simulink library "halin"  (R2021b)
settings: Solver=VariableStepAuto  StartTime=0.0  StopTime=10.0  RelTol=1e-3
undefined symbols (not defined in the file): KHAL_CAN1ABM1E2E_flg, KHAL_CAN1ESC1E2E_flg, KHAL_CAN1ESC5E2E_flg, KHAL_CAN1ESC7E2E_flg, KHAL_CAN1FCM2E2E_flg, KHAL_CAN1FCM3E2E_flg, KHAL_CAN1FCM4E2E_flg, KHAL_CAN3BMS1E2E_flg, KHAL_CAN3BMS6E2E_flg, KHAL_CAN3CCU1E2E_flg, KHAL_CAN3CCU2E2E_flg, KHAL_CAN3MCUF1E2E_flg, KHAL_CAN3MCUR1E2E_flg, KHAL_CAN3Shifter1E2E_flg, TRUE
libraries: simulink x420, FVT_lib x149, hcu_lib x49
(part 5 of 14)

== system halin/HAL_IN/CAN1/ESC1 ==
  DT_CAN1_SG_ESC1 : Inport
  0x5f : Constant  Value=0x5f
  0xb3 : Constant  Value=0xb3
  BitwiseAND{,1..9} (10 alike) : simulink/Logic and Bit Operations/Bitwise Operator  logicop=AND  UseBitMask=on  BitMask=0xFF  BitMaskRealWorld=Stored Integer
  BitwiseOR : simulink/Logic and Bit Operations/Bitwise Operator  logicop=OR  UseBitMask=off  NumInputPorts=2  BitMask=bin2dec('11011001')  BitMaskRealWorld=Stored Integer
  BitwiseOR1 : simulink/Logic and Bit Operations/Bitwise Operator  logicop=OR  UseBitMask=off  NumInputPorts=3  BitMask=bin2dec('11011001')  BitMaskRealWorld=Stored Integer
  BitwiseOR{2..6} (5 alike) : simulink/Logic and Bit Operations/Bitwise Operator  logicop=OR  UseBitMask=off  BitMask=bin2dec('11011001')  BitMaskRealWorld=Stored Integer
  DDM_ESC_CS&RC_Comparison : FVT_lib/hal/DDM_ESC_CS&RC_Comparison  MsgCycleTime=10
  Data Type Conversion{,1..9} (10 alike) : DataTypeConversion  OutDataTypeStr=uint8
  ESC1CS : Subsystem
  ESC1RC : Subsystem
  FrPTCSActive : Subsystem
  FrntAxlTrqReqDrv : Subsystem
  KHAL_CAN1ESC1E2E_flg : Constant  Value=KHAL_CAN1ESC1E2E_flg
  LeftShift : ArithShift  BitShiftNumber=4  BitShiftDirection=Left
  LeftShift1 : ArithShift  BitShiftDirection=Left
  LeftShift2 : ArithShift  BitShiftNumber=5  BitShiftDirection=Left
  LeftShift3 : ArithShift  BitShiftNumber=6  BitShiftDirection=Left
  MessageRollingCounter : FVT_lib/hal/MessageRollingCounter  CounterMAX=14  task_time_ms=5  msg_time_ms=10
  Mux : Mux  Inputs=8
  RearAxlTrqReqDrv : Subsystem
  RightShift : ArithShift  BitShiftNumber=8
  RightShift1 : ArithShift
  RightShift2 : ArithShift  BitShiftNumber=8
  RightShift3 : ArithShift
  RightShift4 : ArithShift  BitShiftNumber=8
  RightShift5 : ArithShift
  RrPTCSActive : Subsystem
  VehSpeed : Subsystem
  bus_selector : BusSelector  OutputSignals=CAN1_ESC1_CS,CAN1_ESC1_RC,CAN1_Fr_PTCS_Active,CAN1_FrntAxlTrqReq_Drv,CAN1_RearAxlTrqReq_Drv,CAN1_Rr_PTCS_Active,CAN1_VehSpeed
  bus_selector1 : BusSelector  OutputSignals=CAN1_ESC1_CS
  bus_selector2 : BusSelector  OutputSignals=CAN1_ESC1_RC
  bus_selector3 : BusSelector  OutputSignals=CAN1_Fr_PTCS_Active
  bus_selector4 : BusSelector  OutputSignals=CAN1_FrntAxlTrqReq_Drv
  bus_selector5 : BusSelector  OutputSignals=CAN1_RearAxlTrqReq_Drv
  bus_selector6 : BusSelector  OutputSignals=CAN1_Rr_PTCS_Active
  bus_selector7 : BusSelector  OutputSignals=CAN1_VehSpeed
  constant : Constant  Value=0x0  OutDataTypeStr=uint8
  VHAL_ESC1CSErr_flg : Outport
  VHAL_ESC1RCErr_flg : Outport  Port=2
  VHAL_ESC1CS_enum : Outport  Port=3
  VHAL_ESC1RC_enum : Outport  Port=4
  VHAL_FrPTCSActive_flg : Outport  Port=5
  VHAL_FrntAxlTrqReqDrv_Nm : Outport  Port=6
  VHAL_RearAxlTrqReqDrv_Nm : Outport  Port=7
  VHAL_RrPTCSActive_flg : Outport  Port=8
  VHAL_VehSpeed_kph : Outport  Port=9
  wires:
  DT_CAN1_SG_ESC1/1 -> [DT_CAN1_SG_ESC1]
  [DT_CAN1_SG_ESC1] -> bus_selector/1
  bus_selector/1 -> [CAN1_ESC1_CS]  "<CAN1_ESC1_CS>"
  [CAN1_ESC1_CS] -> LeftShift/1
  LeftShift/1 -> BitwiseAND/1
  BitwiseAND/1 -> [Byte_0_CAN1_ESC1_CS]
  bus_selector/2 -> [CAN1_ESC1_RC]  "<CAN1_ESC1_RC>"
  [CAN1_ESC1_RC] -> LeftShift1/1
  LeftShift1/1 -> BitwiseAND1/1
  BitwiseAND1/1 -> [Byte_0_CAN1_ESC1_RC]
  bus_selector/3 -> [CAN1_Fr_PTCS_Active]  "<CAN1_Fr_PTCS_Active>"
  [CAN1_Fr_PTCS_Active] -> LeftShift2/1
  LeftShift2/1 -> BitwiseAND2/1
  BitwiseAND2/1 -> [Byte_2_CAN1_Fr_PTCS_Active]
  bus_selector/4 -> [CAN1_FrntAxlTrqReq_Drv]  "<CAN1_FrntAxlTrqReq_Drv>"
  [CAN1_FrntAxlTrqReq_Drv] -> RightShift/1, RightShift1/1
  RightShift/1 -> BitwiseAND3/1
  BitwiseAND3/1 -> [Byte_4_CAN1_FrntAxlTrqReq_Drv]
  RightShift1/1 -> BitwiseAND4/1
  BitwiseAND4/1 -> [Byte_5_CAN1_FrntAxlTrqReq_Drv]
  bus_selector/5 -> [CAN1_RearAxlTrqReq_Drv]  "<CAN1_RearAxlTrqReq_Drv>"
  [CAN1_RearAxlTrqReq_Drv] -> RightShift2/1, RightShift3/1
  RightShift2/1 -> BitwiseAND5/1
  BitwiseAND5/1 -> [Byte_6_CAN1_RearAxlTrqReq_Drv]
  RightShift3/1 -> BitwiseAND6/1
  BitwiseAND6/1 -> [Byte_7_CAN1_RearAxlTrqReq_Drv]
  bus_selector/6 -> [CAN1_Rr_PTCS_Active]  "<CAN1_Rr_PTCS_Active>"
  [CAN1_Rr_PTCS_Active] -> LeftShift3/1
  LeftShift3/1 -> BitwiseAND7/1
  BitwiseAND7/1 -> [Byte_2_CAN1_Rr_PTCS_Active]
  bus_selector/7 -> [CAN1_VehSpeed]  "<CAN1_VehSpeed>"
  [CAN1_VehSpeed] -> RightShift4/1, RightShift5/1
  RightShift4/1 -> BitwiseAND8/1
  BitwiseAND8/1 -> [Byte_2_CAN1_VehSpeed]
  RightShift5/1 -> BitwiseAND9/1
  BitwiseAND9/1 -> [Byte_3_CAN1_VehSpeed]
  Data Type Conversion/1 -> BitwiseOR/1
  [Byte_0_CAN1_ESC1_CS] -> Data Type Conversion/1
  Data Type Conversion1/1 -> BitwiseOR/2
  [Byte_0_CAN1_ESC1_RC] -> Data Type Conversion1/1
  BitwiseOR/1 -> [Byte_0]
  constant/1 -> [Byte_1]
  Data Type Conversion2/1 -> BitwiseOR1/1
  [Byte_2_CAN1_Fr_PTCS_Active] -> Data Type Conversion2/1
  Data Type Conversion3/1 -> BitwiseOR1/2
  [Byte_2_CAN1_Rr_PTCS_Active] -> Data Type Conversion3/1
  Data Type Conversion4/1 -> BitwiseOR1/3
  [Byte_2_CAN1_VehSpeed] -> Data Type Conversion4/1
  BitwiseOR1/1 -> [Byte_2]
  Data Type Conversion5/1 -> BitwiseOR2/1
  [Byte_3_CAN1_VehSpeed] -> Data Type Conversion5/1
  BitwiseOR2/1 -> [Byte_3]
  Data Type Conversion6/1 -> BitwiseOR3/1
  [Byte_4_CAN1_FrntAxlTrqReq_Drv] -> Data Type Conversion6/1
  BitwiseOR3/1 -> [Byte_4]
  Data Type Conversion7/1 -> BitwiseOR4/1
  [Byte_5_CAN1_FrntAxlTrqReq_Drv] -> Data Type Conversion7/1
  BitwiseOR4/1 -> [Byte_5]
  Data Type Conversion8/1 -> BitwiseOR5/1
  [Byte_6_CAN1_RearAxlTrqReq_Drv] -> Data Type Conversion8/1
  BitwiseOR5/1 -> [Byte_6]
  Data Type Conversion9/1 -> BitwiseOR6/1
  [Byte_7_CAN1_RearAxlTrqReq_Drv] -> Data Type Conversion9/1
  BitwiseOR6/1 -> [Byte_7]
  [Byte_0] -> Mux/1
  [Byte_1] -> Mux/2
  [Byte_2] -> Mux/3
  [Byte_3] -> Mux/4
  [Byte_4] -> Mux/5
  [Byte_5] -> Mux/6
  [Byte_6] -> Mux/7
  [Byte_7] -> Mux/8
  Mux/1 -> [VHAL_CAN1ESC1_raw]
  KHAL_CAN1ESC1E2E_flg/1 -> DDM_ESC_CS&RC_Comparison/1
  0xb3/1 -> DDM_ESC_CS&RC_Comparison/2
  0x5f/1 -> DDM_ESC_CS&RC_Comparison/3
  [VHAL_CAN1ESC1_raw] -> DDM_ESC_CS&RC_Comparison/4
  [RC_ECU] -> DDM_ESC_CS&RC_Comparison/5
  MessageRollingCounter/1 -> DDM_ESC_CS&RC_Comparison/6
  DDM_ESC_CS&RC_Comparison/1 -> VHAL_ESC1CSErr_flg/1
  DDM_ESC_CS&RC_Comparison/2 -> VHAL_ESC1RCErr_flg/1
  [DT_CAN1_SG_ESC1] -> bus_selector1/1
  bus_selector1/1 -> ESC1CS/1(ESC1_CS)  "<CAN1_ESC1_CS>"
  ESC1CS/1(VHAL_ESC1CS_enum) -> VHAL_ESC1CS_enum/1
  [DT_CAN1_SG_ESC1] -> bus_selector2/1
  bus_selector2/1 -> ESC1RC/1(ESC1_RC)  "<CAN1_ESC1_RC>"
  ESC1RC/1(VHAL_ESC1RC_enum) -> VHAL_ESC1RC_enum/1, [RC_ECU]
  [DT_CAN1_SG_ESC1] -> bus_selector3/1
  bus_selector3/1 -> FrPTCSActive/1(Fr_PTCS_Active)  "<CAN1_Fr_PTCS_Active>"
  FrPTCSActive/1(VHAL_FrPTCSActive_flg) -> VHAL_FrPTCSActive_flg/1
  [DT_CAN1_SG_ESC1] -> bus_selector4/1
  bus_selector4/1 -> FrntAxlTrqReqDrv/1(FrntAxlTrqReq_Drv)  "<CAN1_FrntAxlTrqReq_Drv>"
  FrntAxlTrqReqDrv/1(VHAL_FrntAxlTrqReqDrv_Nm) -> VHAL_FrntAxlTrqReqDrv_Nm/1
  [DT_CAN1_SG_ESC1] -> bus_selector5/1
  bus_selector5/1 -> RearAxlTrqReqDrv/1(RearAxlTrqReq_Drv)  "<CAN1_RearAxlTrqReq_Drv>"
  RearAxlTrqReqDrv/1(VHAL_RearAxlTrqReqDrv_Nm) -> VHAL_RearAxlTrqReqDrv_Nm/1
  [DT_CAN1_SG_ESC1] -> bus_selector6/1
  bus_selector6/1 -> RrPTCSActive/1(Rr_PTCS_Active)  "<CAN1_Rr_PTCS_Active>"
  RrPTCSActive/1(VHAL_RrPTCSActive_flg) -> VHAL_RrPTCSActive_flg/1
  [DT_CAN1_SG_ESC1] -> bus_selector7/1
  bus_selector7/1 -> VehSpeed/1(VehSpeed)  "<CAN1_VehSpeed>"
  VehSpeed/1(VHAL_VehSpeed_kph) -> VHAL_VehSpeed_kph/1

== system halin/HAL_IN/CAN1/ESC2 ==
  DT_CAN1_SG_ESC2 : Inport
  LFPulseCount : Subsystem
  LFPulseCountV : Subsystem
  LFRawWhlSpeed : Subsystem
  LFRawWhlSpeedV : Subsystem
  LFWhlRotDir : Subsystem
  RFPulseCount : Subsystem
  RFPulseCountV : Subsystem
  RFRawWhlSpeed : Subsystem
  RFRawWhlSpeedV : Subsystem
  RFWhlRotDir : Subsystem
  bus_selector : BusSelector  OutputSignals=CAN1_LF_PulseCount
  bus_selector1 : BusSelector  OutputSignals=CAN1_LF_PulseCount_V
  bus_selector2 : BusSelector  OutputSignals=CAN1_LF_RawWhlSpeed
  bus_selector3 : BusSelector  OutputSignals=CAN1_LF_RawWhlSpeed_V
  bus_selector4 : BusSelector  OutputSignals=CAN1_LF_WhlRotDir
  bus_selector5 : BusSelector  OutputSignals=CAN1_RF_PulseCount
  bus_selector6 : BusSelector  OutputSignals=CAN1_RF_PulseCount_V
  bus_selector7 : BusSelector  OutputSignals=CAN1_RF_RawWhlSpeed
  bus_selector8 : BusSelector  OutputSignals=CAN1_RF_RawWhlSpeed_V
  bus_selector9 : BusSelector  OutputSignals=CAN1_RF_WhlRotDir
  VHAL_LFPulseCount_enum : Outport
  VHAL_LFPulseCountV_flg : Outport  Port=2
  VHAL_LFRawWhlSpeed_kph : Outport  Port=3
  VHAL_LFRawWhlSpeedV_flg : Outport  Port=4
  VHAL_LFWhlRotDir_enum : Outport  Port=5
  VHAL_RFPulseCount_enum : Outport  Port=6
  VHAL_RFPulseCountV_flg : Outport  Port=7
  VHAL_RFRawWhlSpeed_kph : Outport  Port=8
  VHAL_RFRawWhlSpeedV_flg : Outport  Port=9
  VHAL_RFWhlRotDir_enum : Outport  Port=10
  wires:
  DT_CAN1_SG_ESC2/1 -> [DT_CAN1_SG_ESC2]
  [DT_CAN1_SG_ESC2] -> bus_selector/1
  bus_selector/1 -> LFPulseCount/1(LF_PulseCount)  "<CAN1_LF_PulseCount>"
  LFPulseCount/1(VHAL_LFPulseCount_enum) -> VHAL_LFPulseCount_enum/1
  [DT_CAN1_SG_ESC2] -> bus_selector1/1
  bus_selector1/1 -> LFPulseCountV/1(LF_PulseCount_V)  "<CAN1_LF_PulseCount_V>"
  LFPulseCountV/1(VHAL_LFPulseCountV_flg) -> VHAL_LFPulseCountV_flg/1
  [DT_CAN1_SG_ESC2] -> bus_selector2/1
  bus_selector2/1 -> LFRawWhlSpeed/1(LF_RawWhlSpeed)  "<CAN1_LF_RawWhlSpeed>"
  LFRawWhlSpeed/1(VHAL_LFRawWhlSpeed_kph) -> VHAL_LFRawWhlSpeed_kph/1
  [DT_CAN1_SG_ESC2] -> bus_selector3/1
  bus_selector3/1 -> LFRawWhlSpeedV/1(LF_RawWhlSpeed_V)  "<CAN1_LF_RawWhlSpeed_V>"
  LFRawWhlSpeedV/1(VHAL_LFRawWhlSpeedV_flg) -> VHAL_LFRawWhlSpeedV_flg/1
  [DT_CAN1_SG_ESC2] -> bus_selector4/1
  bus_selector4/1 -> LFWhlRotDir/1(LF_WhlRotDir)  "<CAN1_LF_WhlRotDir>"
  LFWhlRotDir/1(VHAL_LFWhlRotDir_enum) -> VHAL_LFWhlRotDir_enum/1
  [DT_CAN1_SG_ESC2] -> bus_selector5/1
  bus_selector5/1 -> RFPulseCount/1(RF_PulseCount)  "<CAN1_RF_PulseCount>"
  RFPulseCount/1(VHAL_RFPulseCount_enum) -> VHAL_RFPulseCount_enum/1
  [DT_CAN1_SG_ESC2] -> bus_selector6/1
  bus_selector6/1 -> RFPulseCountV/1(RF_PulseCount_V)  "<CAN1_RF_PulseCount_V>"
  RFPulseCountV/1(VHAL_RFPulseCountV_flg) -> VHAL_RFPulseCountV_flg/1
  [DT_CAN1_SG_ESC2] -> bus_selector7/1
  bus_selector7/1 -> RFRawWhlSpeed/1(RF_RawWhlSpeed)  "<CAN1_RF_RawWhlSpeed>"
  RFRawWhlSpeed/1(VHAL_RFRawWhlSpeed_kph) -> VHAL_RFRawWhlSpeed_kph/1
  [DT_CAN1_SG_ESC2] -> bus_selector8/1
  bus_selector8/1 -> RFRawWhlSpeedV/1(RF_RawWhlSpeed_V)  "<CAN1_RF_RawWhlSpeed_V>"
  RFRawWhlSpeedV/1(VHAL_RFRawWhlSpeedV_flg) -> VHAL_RFRawWhlSpeedV_flg/1
  [DT_CAN1_SG_ESC2] -> bus_selector9/1
  bus_selector9/1 -> RFWhlRotDir/1(RF_WhlRotDir)  "<CAN1_RF_WhlRotDir>"
  RFWhlRotDir/1(VHAL_RFWhlRotDir_enum) -> VHAL_RFWhlRotDir_enum/1

== system halin/HAL_IN/CAN1/ESC3 ==
  DT_CAN1_SG_ESC3 : Inport
  LRPulseCount : Subsystem
  LRPulseCountV : Subsystem
  LRRawWhlSpeed : Subsystem
  LRRawWhlSpeedV : Subsystem
  LRWhlRotDir : Subsystem
  RRPulseCount : Subsystem
  RRPulseCountV : Subsystem
  RRRawWhlSpeed : Subsystem
  RRRawWhlSpeedV : Subsystem
  RRWhlRotDir : Subsystem
  bus_selector : BusSelector  OutputSignals=CAN1_LR_PulseCount
  bus_selector1 : BusSelector  OutputSignals=CAN1_LR_PulseCount_V
  bus_selector2 : BusSelector  OutputSignals=CAN1_LR_RawWhlSpeed
  bus_selector3 : BusSelector  OutputSignals=CAN1_LR_RawWhlSpeed_V
  bus_selector4 : BusSelector  OutputSignals=CAN1_LR_WhlRotDir
  bus_selector5 : BusSelector  OutputSignals=CAN1_RR_PulseCount
  bus_selector6 : BusSelector  OutputSignals=CAN1_RR_PulseCount_V
  bus_selector7 : BusSelector  OutputSignals=CAN1_RR_RawWhlSpeed
  bus_selector8 : BusSelector  OutputSignals=CAN1_RR_RawWhlSpeed_V
  bus_selector9 : BusSelector  OutputSignals=CAN1_RR_WhlRotDir
  VHAL_LRPulseCount_enum : Outport
  VHAL_LRPulseCountV_flg : Outport  Port=2
  VHAL_LRRawWhlSpeed_kph : Outport  Port=3
  VHAL_LRRawWhlSpeedV_flg : Outport  Port=4
  VHAL_LRWhlRotDir_enum : Outport  Port=5
  VHAL_RRPulseCount_enum : Outport  Port=6
  VHAL_RRPulseCountV_flg : Outport  Port=7
  VHAL_RRRawWhlSpeed_kph : Outport  Port=8
  VHAL_RRRawWhlSpeedV_flg : Outport  Port=9
  VHAL_RRWhlRotDir_enum : Outport  Port=10
  wires:
  DT_CAN1_SG_ESC3/1 -> [DT_CAN1_SG_ESC3]
  [DT_CAN1_SG_ESC3] -> bus_selector/1
  bus_selector/1 -> LRPulseCount/1(LR_PulseCount)  "<CAN1_LR_PulseCount>"
  LRPulseCount/1(VHAL_LRPulseCount_enum) -> VHAL_LRPulseCount_enum/1
  [DT_CAN1_SG_ESC3] -> bus_selector1/1
  bus_selector1/1 -> LRPulseCountV/1(LR_PulseCount_V)  "<CAN1_LR_PulseCount_V>"
  LRPulseCountV/1(VHAL_LRPulseCountV_flg) -> VHAL_LRPulseCountV_flg/1
  [DT_CAN1_SG_ESC3] -> bus_selector2/1
  bus_selector2/1 -> LRRawWhlSpeed/1(LR_RawWhlSpeed)  "<CAN1_LR_RawWhlSpeed>"
  LRRawWhlSpeed/1(VHAL_LRRawWhlSpeed_kph) -> VHAL_LRRawWhlSpeed_kph/1
  [DT_CAN1_SG_ESC3] -> bus_selector3/1
  bus_selector3/1 -> LRRawWhlSpeedV/1(LR_RawWhlSpeed_V)  "<CAN1_LR_RawWhlSpeed_V>"
  LRRawWhlSpeedV/1(VHAL_LRRawWhlSpeedV_flg) -> VHAL_LRRawWhlSpeedV_flg/1
  [DT_CAN1_SG_ESC3] -> bus_selector4/1
  bus_selector4/1 -> LRWhlRotDir/1(LR_WhlRotDir)  "<CAN1_LR_WhlRotDir>"
  LRWhlRotDir/1(VHAL_LRWhlRotDir_enum) -> VHAL_LRWhlRotDir_enum/1
  [DT_CAN1_SG_ESC3] -> bus_selector5/1
  bus_selector5/1 -> RRPulseCount/1(RR_PulseCount)  "<CAN1_RR_PulseCount>"
  RRPulseCount/1(VHAL_RRPulseCount_enum) -> VHAL_RRPulseCount_enum/1
  [DT_CAN1_SG_ESC3] -> bus_selector6/1
  bus_selector6/1 -> RRPulseCountV/1(RR_PulseCount_V)  "<CAN1_RR_PulseCount_V>"
  RRPulseCountV/1(VHAL_RRPulseCountV_flg) -> VHAL_RRPulseCountV_flg/1
  [DT_CAN1_SG_ESC3] -> bus_selector7/1
  bus_selector7/1 -> RRRawWhlSpeed/1(RR_RawWhlSpeed)  "<CAN1_RR_RawWhlSpeed>"
  RRRawWhlSpeed/1(VHAL_RRRawWhlSpeed_kph) -> VHAL_RRRawWhlSpeed_kph/1
  [DT_CAN1_SG_ESC3] -> bus_selector8/1
  bus_selector8/1 -> RRRawWhlSpeedV/1(RR_RawWhlSpeed_V)  "<CAN1_RR_RawWhlSpeed_V>"
  RRRawWhlSpeedV/1(VHAL_RRRawWhlSpeedV_flg) -> VHAL_RRRawWhlSpeedV_flg/1
  [DT_CAN1_SG_ESC3] -> bus_selector9/1
  bus_selector9/1 -> RRWhlRotDir/1(RR_WhlRotDir)  "<CAN1_RR_WhlRotDir>"
  RRWhlRotDir/1(VHAL_RRWhlRotDir_enum) -> VHAL_RRWhlRotDir_enum/1

== system halin/HAL_IN/CAN1/ESC4 ==
  DT_CAN1_SG_ESC4 : Inport
  ABSActive : Subsystem
  ABSFailed : Subsystem
  AVHActive : Subsystem
  AVHFailed : Subsystem
  BTCSActive : Subsystem
  EBDActive : Subsystem
  EBDFailed : Subsystem
  ESCActive : Subsystem
  ESCFailed : Subsystem
  ESSActive : Subsystem
  GRADE : Subsystem
  HBBActive : Subsystem
  HBBFailed : Subsystem
  HDDActive : Subsystem
  HDDFailed : Subsystem
  HSAActive : Subsystem
  HSAFailed : Subsystem
  PBAFailed : Subsystem
  TCSActive : Subsystem
  TCSFailed : Subsystem
  bus_selector : BusSelector  OutputSignals=CAN1_ABS_Active
  bus_selector1 : BusSelector  OutputSignals=CAN1_ABS_Failed
  bus_selector10 : BusSelector  OutputSignals=CAN1_GRADE
  bus_selector11 : BusSelector  OutputSignals=CAN1_HBB_Active
  bus_selector12 : BusSelector  OutputSignals=CAN1_HBB_Failed
  bus_selector13 : BusSelector  OutputSignals=CAN1_HDD_Active
  bus_selector14 : BusSelector  OutputSignals=CAN1_HDD_Failed
  bus_selector15 : BusSelector  OutputSignals=CAN1_HSA_Active
  bus_selector16 : BusSelector  OutputSignals=CAN1_HSA_Failed
  bus_selector17 : BusSelector  OutputSignals=CAN1_PBA_Failed
  bus_selector18 : BusSelector  OutputSignals=CAN1_TCS_Active
  bus_selector19 : BusSelector  OutputSignals=CAN1_TCS_Failed
  bus_selector2 : BusSelector  OutputSignals=CAN1_AVH_Active
  bus_selector3 : BusSelector  OutputSignals=CAN1_AVH_Failed
  bus_selector4 : BusSelector  OutputSignals=CAN1_BTCS_Active
  bus_selector5 : BusSelector  OutputSignals=CAN1_EBD_Active
  bus_selector6 : BusSelector  OutputSignals=CAN1_EBD_Failed
  bus_selector7 : BusSelector  OutputSignals=CAN1_ESC_Active
  bus_selector8 : BusSelector  OutputSignals=CAN1_ESC_Failed
  bus_selector9 : BusSelector  OutputSignals=CAN1_ESS_Active
  VHAL_ABSActive_flg : Outport
  VHAL_ABSFailed_flg : Outport  Port=2
  VHAL_AVHActive_flg : Outport  Port=3
  VHAL_AVHFailed_flg : Outport  Port=4
  VHAL_BTCSActive_flg : Outport  Port=5
  VHAL_EBDActive_flg : Outport  Port=6
  VHAL_EBDFailed_flg : Outport  Port=7
  VHAL_ESCActive_flg : Outport  Port=8
  VHAL_ESCFailed_flg : Outport  Port=9
  VHAL_ESSActive_flg : Outport  Port=10
  VHAL_GRADE_Deg : Outport  Port=11
  VHAL_HBBActive_flg : Outport  Port=12
  VHAL_HBBFailed_flg : Outport  Port=13
  VHAL_HDDActive_flg : Outport  Port=14
  VHAL_HDDFailed_flg : Outport  Port=15
  VHAL_HSAActive_flg : Outport  Port=16
  VHAL_HSAFailed_flg : Outport  Port=17
  VHAL_PBAFailed_flg : Outport  Port=18
  VHAL_TCSActive_flg : Outport  Port=19
  VHAL_TCSFailed_flg : Outport  Port=20
  wires:
  DT_CAN1_SG_ESC4/1 -> [DT_CAN1_SG_ESC4]
  [DT_CAN1_SG_ESC4] -> bus_selector/1
  bus_selector/1 -> ABSActive/1(ABS_Active)  "<CAN1_ABS_Active>"
  ABSActive/1(VHAL_ABSActive_flg) -> VHAL_ABSActive_flg/1
  [DT_CAN1_SG_ESC4] -> bus_selector1/1
  bus_selector1/1 -> ABSFailed/1(ABS_Failed)  "<CAN1_ABS_Failed>"
  ABSFailed/1(VHAL_ABSFailed_flg) -> VHAL_ABSFailed_flg/1
  [DT_CAN1_SG_ESC4] -> bus_selector2/1
  bus_selector2/1 -> AVHActive/1(AVH_Active)  "<CAN1_AVH_Active>"
  AVHActive/1(VHAL_AVHActive_flg) -> VHAL_AVHActive_flg/1
  [DT_CAN1_SG_ESC4] -> bus_selector3/1
  bus_selector3/1 -> AVHFailed/1(AVH_Failed)  "<CAN1_AVH_Failed>"
  AVHFailed/1(VHAL_AVHFailed_flg) -> VHAL_AVHFailed_flg/1
  [DT_CAN1_SG_ESC4] -> bus_selector4/1
  bus_selector4/1 -> BTCSActive/1(BTCS_Active)  "<CAN1_BTCS_Active>"
  BTCSActive/1(VHAL_BTCSActive_flg) -> VHAL_BTCSActive_flg/1
  [DT_CAN1_SG_ESC4] -> bus_selector5/1
  bus_selector5/1 -> EBDActive/1(EBD_Active)  "<CAN1_EBD_Active>"
  EBDActive/1(VHAL_EBDActive_flg) -> VHAL_EBDActive_flg/1
  [DT_CAN1_SG_ESC4] -> bus_selector6/1
  bus_selector6/1 -> EBDFailed/1(EBD_Failed)  "<CAN1_EBD_Failed>"
  EBDFailed/1(VHAL_EBDFailed_flg) -> VHAL_EBDFailed_flg/1
  [DT_CAN1_SG_ESC4] -> bus_selector7/1
  bus_selector7/1 -> ESCActive/1(ESC_Active)  "<CAN1_ESC_Active>"
  ESCActive/1(VHAL_ESCActive_flg) -> VHAL_ESCActive_flg/1
  [DT_CAN1_SG_ESC4] -> bus_selector8/1
  bus_selector8/1 -> ESCFailed/1(ESC_Failed)  "<CAN1_ESC_Failed>"
  ESCFailed/1(VHAL_ESCFailed_flg) -> VHAL_ESCFailed_flg/1
  [DT_CAN1_SG_ESC4] -> bus_selector9/1
  bus_selector9/1 -> ESSActive/1(ESS_Active)  "<CAN1_ESS_Active>"
  ESSActive/1(VHAL_ESSActive_flg) -> VHAL_ESSActive_flg/1
  [DT_CAN1_SG_ESC4] -> bus_selector10/1
  bus_selector10/1 -> GRADE/1(GRADE)  "<CAN1_GRADE>"
  GRADE/1(VHAL_GRADE_Deg) -> VHAL_GRADE_Deg/1
  [DT_CAN1_SG_ESC4] -> bus_selector11/1
  bus_selector11/1 -> HBBActive/1(HBB_Active)  "<CAN1_HBB_Active>"
  HBBActive/1(VHAL_HBBActive_flg) -> VHAL_HBBActive_flg/1
  [DT_CAN1_SG_ESC4] -> bus_selector12/1
  bus_selector12/1 -> HBBFailed/1(HBB_Failed)  "<CAN1_HBB_Failed>"
  HBBFailed/1(VHAL_HBBFailed_flg) -> VHAL_HBBFailed_flg/1
  [DT_CAN1_SG_ESC4] -> bus_selector13/1
  bus_selector13/1 -> HDDActive/1(HDD_Active)  "<CAN1_HDD_Active>"
  HDDActive/1(VHAL_HDDActive_flg) -> VHAL_HDDActive_flg/1
  [DT_CAN1_SG_ESC4] -> bus_selector14/1
  bus_selector14/1 -> HDDFailed/1(HDD_Failed)  "<CAN1_HDD_Failed>"
  HDDFailed/1(VHAL_HDDFailed_flg) -> VHAL_HDDFailed_flg/1
  [DT_CAN1_SG_ESC4] -> bus_selector15/1
  bus_selector15/1 -> HSAActive/1(HSA_Active)  "<CAN1_HSA_Active>"
  HSAActive/1(VHAL_HSAActive_flg) -> VHAL_HSAActive_flg/1
  [DT_CAN1_SG_ESC4] -> bus_selector16/1
  bus_selector16/1 -> HSAFailed/1(HSA_Failed)  "<CAN1_HSA_Failed>"
  HSAFailed/1(VHAL_HSAFailed_flg) -> VHAL_HSAFailed_flg/1
  [DT_CAN1_SG_ESC4] -> bus_selector17/1
  bus_selector17/1 -> PBAFailed/1(PBA_Failed)  "<CAN1_PBA_Failed>"
  PBAFailed/1(VHAL_PBAFailed_flg) -> VHAL_PBAFailed_flg/1
  [DT_CAN1_SG_ESC4] -> bus_selector18/1
  bus_selector18/1 -> TCSActive/1(TCS_Active)  "<CAN1_TCS_Active>"
  TCSActive/1(VHAL_TCSActive_flg) -> VHAL_TCSActive_flg/1
  [DT_CAN1_SG_ESC4] -> bus_selector19/1
  bus_selector19/1 -> TCSFailed/1(TCS_Failed)  "<CAN1_TCS_Failed>"
  TCSFailed/1(VHAL_TCSFailed_flg) -> VHAL_TCSFailed_flg/1

== system halin/HAL_IN/CAN1/ESC5 ==
  DT_CAN1_SG_ESC5 : Inport
  0x59 : Constant  Value=0x59
  0x6e : Constant  Value=0x6e
  BitwiseAND{,1..13} (14 alike) : simulink/Logic and Bit Operations/Bitwise Operator  logicop=AND  UseBitMask=on  BitMask=0xFF  BitMaskRealWorld=Stored Integer
  BitwiseOR : simulink/Logic and Bit Operations/Bitwise Operator  logicop=OR  UseBitMask=off  NumInputPorts=6  BitMask=bin2dec('11011001')  BitMaskRealWorld=Stored Integer
  BitwiseOR{1,3..7} (6 alike) : simulink/Logic and Bit Operations/Bitwise Operator  logicop=OR  UseBitMask=off  BitMask=bin2dec('11011001')  BitMaskRealWorld=Stored Integer
  BitwiseOR2 : simulink/Logic and Bit Operations/Bitwise Operator  logicop=OR  UseBitMask=off  NumInputPorts=2  BitMask=bin2dec('11011001')  BitMaskRealWorld=Stored Integer
  BrkSwSta : Subsystem
  BrkSwV : Subsystem
  DDM_ESC5_CS&RC_Comparison : FVT_lib/hal/DDM_ESC5_CS&RC_Comparison  MsgCycleTime=10
  Data Type Conversion{,1..13} (14 alike) : DataTypeConversion  OutDataTypeStr=uint8
  ESC5CRC8 : Subsystem
  ESC5RC : Subsystem
  KHAL_CAN1ESC5E2E_flg : Constant  Value=KHAL_CAN1ESC5E2E_flg
  LatAccel : Subsystem
  LatAccelV : Subsystem
  LeftShift : ArithShift  BitShiftNumber=4  BitShiftDirection=Left
  LeftShift1 : ArithShift  BitShiftNumber=5  BitShiftDirection=Left
  LeftShift{2,4,6,9} (4 alike) : ArithShift  BitShiftDirection=Left
  LeftShift3 : ArithShift  BitShiftNumber=4  BitShiftDirection=Left
  LeftShift5 : ArithShift  BitShiftNumber=1  BitShiftDirection=Left
  LeftShift7 : ArithShift  BitShiftNumber=2  BitShiftDirection=Left
  LeftShift8 : ArithShift  BitShiftNumber=3  BitShiftDirection=Left
  LongAccel : Subsystem
  LongAccelV : Subsystem
  MCPressure : Subsystem
  MCPressureV : Subsystem
  MessageRollingCounter : FVT_lib/hal/MessageRollingCounter  CounterMAX=14  task_time_ms=5  msg_time_ms=10
  Mux : Mux  Inputs=7
  RightShift : ArithShift  BitShiftNumber=8
  RightShift1 : ArithShift
  RightShift2 : ArithShift  BitShiftNumber=8
  RightShift3 : ArithShift
  YawRate : Subsystem
  YawRateV : Subsystem
  bus_selector : BusSelector  OutputSignals=CAN1_BrkSw_Sta,CAN1_BrkSw_V,CAN1_ESC5_CRC8,CAN1_ESC5_RC,CAN1_LatAccel,CAN1_LatAccel_V,CAN1_LongAccel,CAN1_LongAccel_V,CAN1_MCPressure,CAN1_MCPressure_V,CAN1_YawRate,CAN1_YawRate_V
  bus_selector1 : BusSelector  OutputSignals=CAN1_BrkSw_Sta
  bus_selector10 : BusSelector  OutputSignals=CAN1_MCPressure_V
  bus_selector11 : BusSelector  OutputSignals=CAN1_YawRate
  bus_selector12 : BusSelector  OutputSignals=CAN1_YawRate_V
  bus_selector2 : BusSelector  OutputSignals=CAN1_BrkSw_V
  bus_selector3 : BusSelector  OutputSignals=CAN1_ESC5_CRC8
  bus_selector4 : BusSelector  OutputSignals=CAN1_ESC5_RC
  bus_selector5 : BusSelector  OutputSignals=CAN1_LatAccel
  bus_selector6 : BusSelector  OutputSignals=CAN1_LatAccel_V
  bus_selector7 : BusSelector  OutputSignals=CAN1_LongAccel
  bus_selector8 : BusSelector  OutputSignals=CAN1_LongAccel_V
  bus_selector9 : BusSelector  OutputSignals=CAN1_MCPressure
  VHAL_ESC5CSErr_flg : Outport
  VHAL_ESC5RCErr_flg : Outport  Port=2
  VHAL_BrkSwSta_flg : Outport  Port=3
  VHAL_BrkSwV_flg : Outport  Port=4
  VHAL_ESC5CRC8_enum : Outport  Port=5
  VHAL_ESC5RC_enum : Outport  Port=6
  VHAL_LatAccel_Gps : Outport  Port=7
  VHAL_LatAccelV_flg : Outport  Port=8
  VHAL_LongAccel_Gps : Outport  Port=9
  VHAL_LongAccelV_flg : Outport  Port=10
  VHAL_MCPressure_bar : Outport  Port=11
  VHAL_MCPressureV_flg : Outport  Port=12
  VHAL_YawRate_degps : Outport  Port=13
  VHAL_YawRateV_flg : Outport  Port=14
  wires:
  DT_CAN1_SG_ESC5/1 -> [DT_CAN1_SG_ESC5]
  [DT_CAN1_SG_ESC5] -> bus_selector/1
  bus_selector/1 -> [CAN1_BrkSw_Sta]  "<CAN1_BrkSw_Sta>"
  [CAN1_BrkSw_Sta] -> LeftShift/1
  LeftShift/1 -> BitwiseAND/1
  BitwiseAND/1 -> [Byte_0_CAN1_BrkSw_Sta]
  bus_selector/2 -> [CAN1_BrkSw_V]  "<CAN1_BrkSw_V>"
  [CAN1_BrkSw_V] -> LeftShift1/1
  LeftShift1/1 -> BitwiseAND1/1
  BitwiseAND1/1 -> [Byte_0_CAN1_BrkSw_V]
  bus_selector/3 -> [CAN1_ESC5_CRC8]  "<CAN1_ESC5_CRC8>"
  [CAN1_ESC5_CRC8] -> LeftShift2/1
  LeftShift2/1 -> BitwiseAND2/1
  BitwiseAND2/1 -> [Byte_1_CAN1_ESC5_CRC8]
  bus_selector/4 -> [CAN1_ESC5_RC]  "<CAN1_ESC5_RC>"
  [CAN1_ESC5_RC] -> LeftShift3/1
  LeftShift3/1 -> BitwiseAND3/1
  BitwiseAND3/1 -> [Byte_2_CAN1_ESC5_RC]
  bus_selector/5 -> [CAN1_LatAccel]  "<CAN1_LatAccel>"
  [CAN1_LatAccel] -> LeftShift4/1
  LeftShift4/1 -> BitwiseAND4/1
  BitwiseAND4/1 -> [Byte_5_CAN1_LatAccel]
  bus_selector/6 -> [CAN1_LatAccel_V]  "<CAN1_LatAccel_V>"
  [CAN1_LatAccel_V] -> LeftShift5/1
  LeftShift5/1 -> BitwiseAND5/1
  BitwiseAND5/1 -> [Byte_0_CAN1_LatAccel_V]
  bus_selector/7 -> [CAN1_LongAccel]  "<CAN1_LongAccel>"
  [CAN1_LongAccel] -> LeftShift6/1
  LeftShift6/1 -> BitwiseAND6/1
  BitwiseAND6/1 -> [Byte_4_CAN1_LongAccel]
  bus_selector/8 -> [CAN1_LongAccel_V]  "<CAN1_LongAccel_V>"
  [CAN1_LongAccel_V] -> LeftShift7/1
  LeftShift7/1 -> BitwiseAND7/1
  BitwiseAND7/1 -> [Byte_0_CAN1_LongAccel_V]
  bus_selector/9 -> [CAN1_MCPressure]  "<CAN1_MCPressure>"
  [CAN1_MCPressure] -> RightShift/1, RightShift1/1
  RightShift/1 -> BitwiseAND8/1
  BitwiseAND8/1 -> [Byte_2_CAN1_MCPressure]
  RightShift1/1 -> BitwiseAND9/1
  BitwiseAND9/1 -> [Byte_3_CAN1_MCPressure]
  bus_selector/10 -> [CAN1_MCPressure_V]  "<CAN1_MCPressure_V>"
  [CAN1_MCPressure_V] -> LeftShift8/1
  LeftShift8/1 -> BitwiseAND10/1
  BitwiseAND10/1 -> [Byte_0_CAN1_MCPressure_V]
  bus_selector/11 -> [CAN1_YawRate]  "<CAN1_YawRate>"
  [CAN1_YawRate] -> RightShift2/1, RightShift3/1
  RightShift2/1 -> BitwiseAND11/1
  BitwiseAND11/1 -> [Byte_6_CAN1_YawRate]
  RightShift3/1 -> BitwiseAND12/1
  BitwiseAND12/1 -> [Byte_7_CAN1_YawRate]
  bus_selector/12 -> [CAN1_YawRate_V]  "<CAN1_YawRate_V>"
  [CAN1_YawRate_V] -> LeftShift9/1
  LeftShift9/1 -> BitwiseAND13/1
  BitwiseAND13/1 -> [Byte_0_CAN1_YawRate_V]
  Data Type Conversion/1 -> BitwiseOR/1
  [Byte_0_CAN1_BrkSw_Sta] -> Data Type Conversion/1
  Data Type Conversion1/1 -> BitwiseOR/2
  [Byte_0_CAN1_BrkSw_V] -> Data Type Conversion1/1
  Data Type Conversion2/1 -> BitwiseOR/3
  [Byte_0_CAN1_LatAccel_V] -> Data Type Conversion2/1
  Data Type Conversion3/1 -> BitwiseOR/4
  [Byte_0_CAN1_LongAccel_V] -> Data Type Conversion3/1
  Data Type Conversion4/1 -> BitwiseOR/5
  [Byte_0_CAN1_MCPressure_V] -> Data Type Conversion4/1
  Data Type Conversion5/1 -> BitwiseOR/6
  [Byte_0_CAN1_YawRate_V] -> Data Type Conversion5/1
  BitwiseOR/1 -> [Byte_0]
  Data Type Conversion6/1 -> BitwiseOR1/1
  [Byte_1_CAN1_ESC5_CRC8] -> Data Type Conversion6/1
  BitwiseOR1/1 -> [Byte_1]
  Data Type Conversion7/1 -> BitwiseOR2/1
  [Byte_2_CAN1_ESC5_RC] -> Data Type Conversion7/1
  Data Type Conversion8/1 -> BitwiseOR2/2
  [Byte_2_CAN1_MCPressure] -> Data Type Conversion8/1
  BitwiseOR2/1 -> [Byte_2]
  Data Type Conversion9/1 -> BitwiseOR3/1
  [Byte_3_CAN1_MCPressure] -> Data Type Conversion9/1
  BitwiseOR3/1 -> [Byte_3]
  Data Type Conversion10/1 -> BitwiseOR4/1
  [Byte_4_CAN1_LongAccel] -> Data Type Conversion10/1
  BitwiseOR4/1 -> [Byte_4]
  Data Type Conversion11/1 -> BitwiseOR5/1
  [Byte_5_CAN1_LatAccel] -> Data Type Conversion11/1
  BitwiseOR5/1 -> [Byte_5]
  Data Type Conversion12/1 -> BitwiseOR6/1
  [Byte_6_CAN1_YawRate] -> Data Type Conversion12/1
  BitwiseOR6/1 -> [Byte_6]
  Data Type Conversion13/1 -> BitwiseOR7/1
  [Byte_7_CAN1_YawRate] -> Data Type Conversion13/1
  BitwiseOR7/1 -> [Byte_7]
  [Byte_0] -> Mux/1
  [Byte_2] -> Mux/2
  [Byte_3] -> Mux/3
  [Byte_4] -> Mux/4
  [Byte_5] -> Mux/5
  [Byte_6] -> Mux/6
  [Byte_7] -> Mux/7
  Mux/1 -> [VHAL_CAN1ESC5noCS_raw]
  KHAL_CAN1ESC5E2E_flg/1 -> DDM_ESC5_CS&RC_Comparison/1
  0x59/1 -> DDM_ESC5_CS&RC_Comparison/2
  0x6e/1 -> DDM_ESC5_CS&RC_Comparison/3
  [VHAL_CAN1ESC5noCS_raw] -> DDM_ESC5_CS&RC_Comparison/4
  [Byte_1] -> DDM_ESC5_CS&RC_Comparison/5
  [RC_ECU] -> DDM_ESC5_CS&RC_Comparison/6
  MessageRollingCounter/1 -> DDM_ESC5_CS&RC_Comparison/7
  DDM_ESC5_CS&RC_Comparison/1 -> VHAL_ESC5CSErr_flg/1
  DDM_ESC5_CS&RC_Comparison/2 -> VHAL_ESC5RCErr_flg/1
  [DT_CAN1_SG_ESC5] -> bus_selector1/1
  bus_selector1/1 -> BrkSwSta/1(BrkSw_Sta)  "<CAN1_BrkSw_Sta>"
  BrkSwSta/1(VHAL_BrkSwSta_flg) -> VHAL_BrkSwSta_flg/1
  [DT_CAN1_SG_ESC5] -> bus_selector2/1
  bus_selector2/1 -> BrkSwV/1(BrkSw_V)  "<CAN1_BrkSw_V>"
  BrkSwV/1(VHAL_BrkSwV_flg) -> VHAL_BrkSwV_flg/1
  [DT_CAN1_SG_ESC5] -> bus_selector3/1
  bus_selector3/1 -> ESC5CRC8/1(ESC5_CRC8)  "<CAN1_ESC5_CRC8>"
  ESC5CRC8/1(VHAL_ESC5CRC8_enum) -> VHAL_ESC5CRC8_enum/1
  [DT_CAN1_SG_ESC5] -> bus_selector4/1
  bus_selector4/1 -> ESC5RC/1(ESC5_RC)  "<CAN1_ESC5_RC>"
  ESC5RC/1(VHAL_ESC5RC_enum) -> VHAL_ESC5RC_enum/1, [RC_ECU]
  [DT_CAN1_SG_ESC5] -> bus_selector5/1
  bus_selector5/1 -> LatAccel/1(LatAccel)  "<CAN1_LatAccel>"
  LatAccel/1(VHAL_LatAccel_Gps) -> VHAL_LatAccel_Gps/1
  [DT_CAN1_SG_ESC5] -> bus_selector6/1
  bus_selector6/1 -> LatAccelV/1(LatAccel_V)  "<CAN1_LatAccel_V>"
  LatAccelV/1(VHAL_LatAccelV_flg) -> VHAL_LatAccelV_flg/1
  [DT_CAN1_SG_ESC5] -> bus_selector7/1
  bus_selector7/1 -> LongAccel/1(LongAccel)  "<CAN1_LongAccel>"
  LongAccel/1(VHAL_LongAccel_Gps) -> VHAL_LongAccel_Gps/1
  [DT_CAN1_SG_ESC5] -> bus_selector8/1
  bus_selector8/1 -> LongAccelV/1(LongAccel_V)  "<CAN1_LongAccel_V>"
  LongAccelV/1(VHAL_LongAccelV_flg) -> VHAL_LongAccelV_flg/1
  [DT_CAN1_SG_ESC5] -> bus_selector9/1
  bus_selector9/1 -> MCPressure/1(MCPressure)  "<CAN1_MCPressure>"
  MCPressure/1(VHAL_MCPressure_bar) -> VHAL_MCPressure_bar/1
  [DT_CAN1_SG_ESC5] -> bus_selector10/1
  bus_selector10/1 -> MCPressureV/1(MCPressure_V)  "<CAN1_MCPressure_V>"
  MCPressureV/1(VHAL_MCPressureV_flg) -> VHAL_MCPressureV_flg/1
  [DT_CAN1_SG_ESC5] -> bus_selector11/1
  bus_selector11/1 -> YawRate/1(YawRate)  "<CAN1_YawRate>"
  YawRate/1(VHAL_YawRate_degps) -> VHAL_YawRate_degps/1
  [DT_CAN1_SG_ESC5] -> bus_selector12/1
  bus_selector12/1 -> YawRateV/1(YawRate_V)  "<CAN1_YawRate_V>"
  YawRateV/1(VHAL_YawRateV_flg) -> VHAL_YawRateV_flg/1

== system halin/HAL_IN/CAN1/ESC6 ==
  DT_CAN1_SG_ESC6 : Inport
  ActBrkLampSta : Subsystem
  ESCADASSta : Subsystem
  ESCAPSSta : Subsystem
  ESCStandstill : Subsystem
  bus_selector : BusSelector  OutputSignals=CAN1_ActBrkLamp_Sta
  bus_selector1 : BusSelector  OutputSignals=CAN1_ESC_ADAS_Sta
  bus_selector2 : BusSelector  OutputSignals=CAN1_ESC_APS_Sta
  bus_selector3 : BusSelector  OutputSignals=CAN1_ESC_Standstill
  VHAL_ActBrkLampSta_flg : Outport
  VHAL_ESCADASSta_enum : Outport  Port=2
  VHAL_ESCAPSSta_enum : Outport  Port=3
  VHAL_ESCStandstill_flg : Outport  Port=4
  wires:
  DT_CAN1_SG_ESC6/1 -> [DT_CAN1_SG_ESC6]
  [DT_CAN1_SG_ESC6] -> bus_selector/1
  bus_selector/1 -> ActBrkLampSta/1(ActBrkLamp_Sta)  "<CAN1_ActBrkLamp_Sta>"
  ActBrkLampSta/1(VHAL_ActBrkLampSta_flg) -> VHAL_ActBrkLampSta_flg/1
  [DT_CAN1_SG_ESC6] -> bus_selector1/1
  bus_selector1/1 -> ESCADASSta/1(ESC_ADAS_Sta)  "<CAN1_ESC_ADAS_Sta>"
  ESCADASSta/1(VHAL_ESCADASSta_enum) -> VHAL_ESCADASSta_enum/1
  [DT_CAN1_SG_ESC6] -> bus_selector2/1
  bus_selector2/1 -> ESCAPSSta/1(ESC_APS_Sta)  "<CAN1_ESC_APS_Sta>"
  ESCAPSSta/1(VHAL_ESCAPSSta_enum) -> VHAL_ESCAPSSta_enum/1
  [DT_CAN1_SG_ESC6] -> bus_selector3/1
  bus_selector3/1 -> ESCStandstill/1(ESC_Standstill)  "<CAN1_ESC_Standstill>"
  ESCStandstill/1(VHAL_ESCStandstill_flg) -> VHAL_ESCStandstill_flg/1

== system halin/HAL_IN/CAN1/ESC7 ==
  DT_CAN1_SG_ESC7 : Inport
  0x4b : Constant  Value=0x4b
  0xc5 : Constant  Value=0xc5
  BitwiseAND{,1..10} (11 alike) : simulink/Logic and Bit Operations/Bitwise Operator  logicop=AND  UseBitMask=on  BitMask=0xFF  BitMaskRealWorld=Stored Integer
  BitwiseOR : simulink/Logic and Bit Operations/Bitwise Operator  logicop=OR  UseBitMask=off  NumInputPorts=2  BitMask=bin2dec('11011001')  BitMaskRealWorld=Stored Integer
  BitwiseOR1 : simulink/Logic and Bit Operations/Bitwise Operator  logicop=OR  UseBitMask=off  NumInputPorts=4  BitMask=bin2dec('11011001')  BitMaskRealWorld=Stored Integer
  BitwiseOR{2..6} (5 alike) : simulink/Logic and Bit Operations/Bitwise Operator  logicop=OR  UseBitMask=off  BitMask=bin2dec('11011001')  BitMaskRealWorld=Stored Integer
  BrkPedalPos : Subsystem
  BrkPedalPosSta : Subsystem
  DDM_ESC_CS&RC_Comparison : FVT_lib/hal/DDM_ESC_CS&RC_Comparison  MsgCycleTime=10
  Data Type Conversion{,1..10} (11 alike) : DataTypeConversion  OutDataTypeStr=uint8
  ESC7CS : Subsystem
  ESC7RC : Subsystem
  FrRBCActive : Subsystem
  FrntAxlTrqReqBrk : Subsystem
  KHAL_CAN1ESC7E2E_flg : Constant  Value=KHAL_CAN1ESC7E2E_flg
  LeftShift : ArithShift  BitShiftDirection=Left
  LeftShift1 : ArithShift  BitShiftDirection=Left
  LeftShift2 : ArithShift  BitShiftNumber=4  BitShiftDirection=Left
  LeftShift3 : ArithShift  BitShiftDirection=Left
  LeftShift4 : ArithShift  BitShiftNumber=4  BitShiftDirection=Left
  LeftShift5 : ArithShift  BitShiftNumber=1  BitShiftDirection=Left
  LeftShift6 : ArithShift  BitShiftNumber=5  BitShiftDirection=Left
  MessageRollingCounter : FVT_lib/hal/MessageRollingCounter  CounterMAX=14  task_time_ms=5  msg_time_ms=10
  Mux : Mux  Inputs=8
  RDCActive : Subsystem
  RearAxlTrqReqBrk : Subsystem
  RightShift : ArithShift  BitShiftNumber=8
  RightShift1 : ArithShift
  RightShift2 : ArithShift  BitShiftNumber=8
  RightShift3 : ArithShift
  RrRBCActive : Subsystem
  bus_selector : BusSelector  OutputSignals=CAN1_BrkPedalPos,CAN1_BrkPedalPos_Sta,CAN1_ESC7_CS,CAN1_ESC7_RC,CAN1_Fr_RBC_Active,CAN1_FrntAxlTrqReq_Brk,CAN1_RDC_Active,CAN1_RearAxlTrqReq_Brk,CAN1_Rr_RBC_Active
  bus_selector1 : BusSelector  OutputSignals=CAN1_BrkPedalPos
  bus_selector2 : BusSelector  OutputSignals=CAN1_BrkPedalPos_Sta
  bus_selector3 : BusSelector  OutputSignals=CAN1_ESC7_CS
  bus_selector4 : BusSelector  OutputSignals=CAN1_ESC7_RC
  bus_selector5 : BusSelector  OutputSignals=CAN1_Fr_RBC_Active
  bus_selector6 : BusSelector  OutputSignals=CAN1_FrntAxlTrqReq_Brk
  bus_selector7 : BusSelector  OutputSignals=CAN1_RDC_Active
  bus_selector8 : BusSelector  OutputSignals=CAN1_RearAxlTrqReq_Brk
  bus_selector9 : BusSelector  OutputSignals=CAN1_Rr_RBC_Active
  constant : Constant  Value=0x0  OutDataTypeStr=uint8
  VHAL_ESC7CSErr_flg : Outport
  VHAL_ESC7RCErr_flg : Outport  Port=2
  VHAL_BrkPedalPos_pct : Outport  Port=3
  VHAL_BrkPedalPosSta_flg : Outport  Port=4
  VHAL_ESC7CS_enum : Outport  Port=5
  VHAL_ESC7RC_enum : Outport  Port=6
  VHAL_FrRBCActive_flg : Outport  Port=7
  VHAL_FrntAxlTrqReqBrk_Nm : Outport  Port=8
  VHAL_RDCActive_enum : Outport  Port=9
  VHAL_RearAxlTrqReqBrk_Nm : Outport  Port=10
  VHAL_RrRBCActive_flg : Outport  Port=11
  wires:
  DT_CAN1_SG_ESC7/1 -> [DT_CAN1_SG_ESC7]
  [DT_CAN1_SG_ESC7] -> bus_selector/1
  bus_selector/1 -> [CAN1_BrkPedalPos]  "<CAN1_BrkPedalPos>"
  [CAN1_BrkPedalPos] -> LeftShift/1
  LeftShift/1 -> BitwiseAND/1
  BitwiseAND/1 -> [Byte_3_CAN1_BrkPedalPos]
  bus_selector/2 -> [CAN1_BrkPedalPos_Sta]  "<CAN1_BrkPedalPos_Sta>"
  [CAN1_BrkPedalPos_Sta] -> LeftShift1/1
  LeftShift1/1 -> BitwiseAND1/1
  BitwiseAND1/1 -> [Byte_2_CAN1_BrkPedalPos_Sta]
  bus_selector/3 -> [CAN1_ESC7_CS]  "<CAN1_ESC7_CS>"
  [CAN1_ESC7_CS] -> LeftShift2/1
  LeftShift2/1 -> BitwiseAND2/1
  BitwiseAND2/1 -> [Byte_0_CAN1_ESC7_CS]
  bus_selector/4 -> [CAN1_ESC7_RC]  "<CAN1_ESC7_RC>"
  [CAN1_ESC7_RC] -> LeftShift3/1
  LeftShift3/1 -> BitwiseAND3/1
  BitwiseAND3/1 -> [Byte_0_CAN1_ESC7_RC]
  bus_selector/5 -> [CAN1_Fr_RBC_Active]  "<CAN1_Fr_RBC_Active>"
  [CAN1_Fr_RBC_Active] -> LeftShift4/1
  LeftShift4/1 -> BitwiseAND4/1
  BitwiseAND4/1 -> [Byte_2_CAN1_Fr_RBC_Active]
  bus_selector/6 -> [CAN1_FrntAxlTrqReq_Brk]  "<CAN1_FrntAxlTrqReq_Brk>"
  [CAN1_FrntAxlTrqReq_Brk] -> RightShift/1, RightShift1/1
  RightShift/1 -> BitwiseAND5/1
  BitwiseAND5/1 -> [Byte_6_CAN1_FrntAxlTrqReq_Brk]
  RightShift1/1 -> BitwiseAND6/1
  BitwiseAND6/1 -> [Byte_7_CAN1_FrntAxlTrqReq_Brk]
  bus_selector/7 -> [CAN1_RDC_Active]  "<CAN1_RDC_Active>"
  [CAN1_RDC_Active] -> LeftShift5/1
  LeftShift5/1 -> BitwiseAND7/1
  BitwiseAND7/1 -> [Byte_2_CAN1_RDC_Active]
  bus_selector/8 -> [CAN1_RearAxlTrqReq_Brk]  "<CAN1_RearAxlTrqReq_Brk>"
  [CAN1_RearAxlTrqReq_Brk] -> RightShift2/1, RightShift3/1
  RightShift2/1 -> BitwiseAND8/1
  BitwiseAND8/1 -> [Byte_4_CAN1_RearAxlTrqReq_Brk]
  RightShift3/1 -> BitwiseAND9/1
  BitwiseAND9/1 -> [Byte_5_CAN1_RearAxlTrqReq_Brk]
  bus_selector/9 -> [CAN1_Rr_RBC_Active]  "<CAN1_Rr_RBC_Active>"
  [CAN1_Rr_RBC_Active] -> LeftShift6/1
  LeftShift6/1 -> BitwiseAND10/1
  BitwiseAND10/1 -> [Byte_2_CAN1_Rr_RBC_Active]
  Data Type Conversion/1 -> BitwiseOR/1
  [Byte_0_CAN1_ESC7_CS] -> Data Type Conversion/1
  Data Type Conversion1/1 -> BitwiseOR/2
  [Byte_0_CAN1_ESC7_RC] -> Data Type Conversion1/1
  BitwiseOR/1 -> [Byte_0]
  constant/1 -> [Byte_1]
  Data Type Conversion2/1 -> BitwiseOR1/1
  [Byte_2_CAN1_BrkPedalPos_Sta] -> Data Type Conversion2/1
  Data Type Conversion3/1 -> BitwiseOR1/2
  [Byte_2_CAN1_Fr_RBC_Active] -> Data Type Conversion3/1
  Data Type Conversion4/1 -> BitwiseOR1/3
  [Byte_2_CAN1_RDC_Active] -> Data Type Conversion4/1
  Data Type Conversion5/1 -> BitwiseOR1/4
  [Byte_2_CAN1_Rr_RBC_Active] -> Data Type Conversion5/1
  BitwiseOR1/1 -> [Byte_2]
  Data Type Conversion6/1 -> BitwiseOR2/1
  [Byte_3_CAN1_BrkPedalPos] -> Data Type Conversion6/1
  BitwiseOR2/1 -> [Byte_3]
  Data Type Conversion7/1 -> BitwiseOR3/1
  [Byte_4_CAN1_RearAxlTrqReq_Brk] -> Data Type Conversion7/1
  BitwiseOR3/1 -> [Byte_4]
  Data Type Conversion8/1 -> BitwiseOR4/1
  [Byte_5_CAN1_RearAxlTrqReq_Brk] -> Data Type Conversion8/1
  BitwiseOR4/1 -> [Byte_5]
  Data Type Conversion9/1 -> BitwiseOR5/1
  [Byte_6_CAN1_FrntAxlTrqReq_Brk] -> Data Type Conversion9/1
  BitwiseOR5/1 -> [Byte_6]
  Data Type Conversion10/1 -> BitwiseOR6/1
  [Byte_7_CAN1_FrntAxlTrqReq_Brk] -> Data Type Conversion10/1
  BitwiseOR6/1 -> [Byte_7]
  [Byte_0] -> Mux/1
  [Byte_1] -> Mux/2
  [Byte_2] -> Mux/3
  [Byte_3] -> Mux/4
  [Byte_4] -> Mux/5
  [Byte_5] -> Mux/6
  [Byte_6] -> Mux/7
  [Byte_7] -> Mux/8
  Mux/1 -> [VHAL_CAN1ESC7_raw]
  KHAL_CAN1ESC7E2E_flg/1 -> DDM_ESC_CS&RC_Comparison/1
  0xc5/1 -> DDM_ESC_CS&RC_Comparison/2
  0x4b/1 -> DDM_ESC_CS&RC_Comparison/3
  [VHAL_CAN1ESC7_raw] -> DDM_ESC_CS&RC_Comparison/4
  [RC_ECU] -> DDM_ESC_CS&RC_Comparison/5
  MessageRollingCounter/1 -> DDM_ESC_CS&RC_Comparison/6
  DDM_ESC_CS&RC_Comparison/1 -> VHAL_ESC7CSErr_flg/1
  DDM_ESC_CS&RC_Comparison/2 -> VHAL_ESC7RCErr_flg/1
  [DT_CAN1_SG_ESC7] -> bus_selector1/1
  bus_selector1/1 -> BrkPedalPos/1(BrkPedalPos)  "<CAN1_BrkPedalPos>"
  BrkPedalPos/1(VHAL_BrkPedalPos_pct) -> VHAL_BrkPedalPos_pct/1
  [DT_CAN1_SG_ESC7] -> bus_selector2/1
  bus_selector2/1 -> BrkPedalPosSta/1(BrkPedalPos_Sta)  "<CAN1_BrkPedalPos_Sta>"
  BrkPedalPosSta/1(VHAL_BrkPedalPosSta_flg) -> VHAL_BrkPedalPosSta_flg/1
  [DT_CAN1_SG_ESC7] -> bus_selector3/1
  bus_selector3/1 -> ESC7CS/1(ESC7_CS)  "<CAN1_ESC7_CS>"
  ESC7CS/1(VHAL_ESC7CS_enum) -> VHAL_ESC7CS_enum/1
  [DT_CAN1_SG_ESC7] -> bus_selector4/1
  bus_selector4/1 -> ESC7RC/1(ESC7_RC)  "<CAN1_ESC7_RC>"
  ESC7RC/1(VHAL_ESC7RC_enum) -> VHAL_ESC7RC_enum/1, [RC_ECU]
  [DT_CAN1_SG_ESC7] -> bus_selector5/1
  bus_selector5/1 -> FrRBCActive/1(Fr_RBC_Active)  "<CAN1_Fr_RBC_Active>"
  FrRBCActive/1(VHAL_FrRBCActive_flg) -> VHAL_FrRBCActive_flg/1
  [DT_CAN1_SG_ESC7] -> bus_selector6/1
  bus_selector6/1 -> FrntAxlTrqReqBrk/1(FrntAxlTrqReq_Brk)  "<CAN1_FrntAxlTrqReq_Brk>"
  FrntAxlTrqReqBrk/1(VHAL_FrntAxlTrqReqBrk_Nm) -> VHAL_FrntAxlTrqReqBrk_Nm/1
  [DT_CAN1_SG_ESC7] -> bus_selector7/1
  bus_selector7/1 -> RDCActive/1(RDC_Active)  "<CAN1_RDC_Active>"
  RDCActive/1(VHAL_RDCActive_enum) -> VHAL_RDCActive_enum/1
  [DT_CAN1_SG_ESC7] -> bus_selector8/1
  bus_selector8/1 -> RearAxlTrqReqBrk/1(RearAxlTrqReq_Brk)  "<CAN1_RearAxlTrqReq_Brk>"
  RearAxlTrqReqBrk/1(VHAL_RearAxlTrqReqBrk_Nm) -> VHAL_RearAxlTrqReqBrk_Nm/1
  [DT_CAN1_SG_ESC7] -> bus_selector9/1
  bus_selector9/1 -> RrRBCActive/1(Rr_RBC_Active)  "<CAN1_Rr_RBC_Active>"
  RrRBCActive/1(VHAL_RrRBCActive_flg) -> VHAL_RrRBCActive_flg/1

== system halin/HAL_IN/CAN1/FCM2 ==
  DT_CAN1_SG_FCM2 : Inport
  0x21 : Constant  Value=0x21
  0xb6 : Constant  Value=0xb6
  ACCRequiredAccel : Subsystem
  ACCVehHoldReq : Subsystem
  BitwiseAND{,1..14} (15 alike) : simulink/Logic and Bit Operations/Bitwise Operator  logicop=AND  UseBitMask=on  BitMask=0xFF  BitMaskRealWorld=Stored Integer
  BitwiseOR : simulink/Logic and Bit Operations/Bitwise Operator  logicop=OR  UseBitMask=off  NumInputPorts=4  BitMask=bin2dec('11011001')  BitMaskRealWorld=Stored Integer
  BitwiseOR1 : simulink/Logic and Bit Operations/Bitwise Operator  logicop=OR  UseBitMask=off  NumInputPorts=3  BitMask=bin2dec('11011001')  BitMaskRealWorld=Stored Integer
  BitwiseOR{2,4,6..7} (4 alike) : simulink/Logic and Bit Operations/Bitwise Operator  logicop=OR  UseBitMask=off  BitMask=bin2dec('11011001')  BitMaskRealWorld=Stored Integer
  BitwiseOR3 : simulink/Logic and Bit Operations/Bitwise Operator  logicop=OR  UseBitMask=off  NumInputPorts=2  BitMask=bin2dec('11011001')  BitMaskRealWorld=Stored Integer
  BitwiseOR5 : simulink/Logic and Bit Operations/Bitwise Operator  logicop=OR  UseBitMask=off  NumInputPorts=2  BitMask=bin2dec('11011001')  BitMaskRealWorld=Stored Integer
  DDM_CS&RC_Comparison : FVT_lib/hal/DDM_CS&RC_Comparison  MsgCycleTime=10
  Data Type Conversion{,1..14} (15 alike) : DataTypeConversion  OutDataTypeStr=uint8
  FCM2Checksum : Subsystem
  FCM2LifeCount : Subsystem
  KHAL_CAN1FCM2E2E_flg : Constant  Value=KHAL_CAN1FCM2E2E_flg
  LeftShift : ArithShift  BitShiftNumber=1  BitShiftDirection=Left
  LeftShift1 : ArithShift  BitShiftNumber=1  BitShiftDirection=Left
  LeftShift2 : ArithShift  BitShiftNumber=7  BitShiftDirection=Left
  LeftShift3 : ArithShift  BitShiftNumber=1  BitShiftDirection=Left
  LeftShift4 : ArithShift  BitShiftNumber=5  BitShiftDirection=Left
  LeftShift5 : ArithShift  BitShiftNumber=3  BitShiftDirection=Left
  LeftShift6 : ArithShift  BitShiftNumber=4  BitShiftDirection=Left
  LeftShift7 : ArithShift  BitShiftDirection=Left
  LeftShift8 : ArithShift  BitShiftNumber=4  BitShiftDirection=Left
  MessageRollingCounter : FVT_lib/hal/MessageRollingCounter  CounterMAX=14  task_time_ms=5  msg_time_ms=10
  Mux : Mux  Inputs=7
  RightShift : ArithShift  BitShiftNumber=8
  RightShift1 : ArithShift
  RightShift2 : ArithShift  BitShiftNumber=8
  RightShift3 : ArithShift
  RightShift4 : ArithShift  BitShiftNumber=8
  RightShift5 : ArithShift
  bus_selector : BusSelector  OutputSignals=CAN1_ACC_ComfortBandLower,CAN1_ACC_ComfortBandUpper,CAN1_ACC_JerkLowerLimit,CAN1_ACC_JerkUpperLimit,CAN1_ACC_RequiredAccel,CAN1_ACC_VehHoldReq,CAN1_ADAS_AEBReq,CAN1_ADAS_DBSReq,CAN1_ADAS_FaultSta,CAN1_AEB_VehHoldReq,CAN1_FCM2_Checksum,CAN1_FCM2_LifeCount
  bus_selector1 : BusSelector  OutputSignals=CAN1_ACC_RequiredAccel
  bus_selector2 : BusSelector  OutputSignals=CAN1_ACC_VehHoldReq
  bus_selector3 : BusSelector  OutputSignals=CAN1_FCM2_Checksum
  bus_selector4 : BusSelector  OutputSignals=CAN1_FCM2_LifeCount
  VHAL_FCM2CSErr_flg : Outport
  VHAL_FCM2RCErr_flg : Outport  Port=2
  VHAL_ACCRequiredAccel_mps2 : Outport  Port=3
  VHAL_ACCVehHoldReq_flg : Outport  Port=4
  VHAL_FCM2Checksum_enum : Outport  Port=5
  VHAL_FCM2LifeCount_enum : Outport  Port=6
  wires:
  DT_CAN1_SG_FCM2/1 -> [DT_CAN1_SG_FCM2]
  [DT_CAN1_SG_FCM2] -> bus_selector/1
  bus_selector/1 -> [CAN1_ACC_ComfortBandLower]  "<CAN1_ACC_ComfortBandLower>"
  [CAN1_ACC_ComfortBandLower] -> RightShift/1, RightShift1/1
  RightShift/1 -> BitwiseAND/1
  BitwiseAND/1 -> [Byte_5_CAN1_ACC_ComfortBandLower]
  RightShift1/1 -> BitwiseAND1/1
  BitwiseAND1/1 -> [Byte_6_CAN1_ACC_ComfortBandLower]
  bus_selector/2 -> [CAN1_ACC_ComfortBandUpper]  "<CAN1_ACC_ComfortBandUpper>"
  [CAN1_ACC_ComfortBandUpper] -> RightShift2/1, RightShift3/1
  RightShift2/1 -> BitwiseAND2/1
  BitwiseAND2/1 -> [Byte_3_CAN1_ACC_ComfortBandUpper]
  RightShift3/1 -> BitwiseAND3/1
  BitwiseAND3/1 -> [Byte_4_CAN1_ACC_ComfortBandUpper]
  bus_selector/3 -> [CAN1_ACC_JerkLowerLimit]  "<CAN1_ACC_JerkLowerLimit>"
  [CAN1_ACC_JerkLowerLimit] -> LeftShift/1
  LeftShift/1 -> BitwiseAND4/1
  BitwiseAND4/1 -> [Byte_5_CAN1_ACC_JerkLowerLimit]
  bus_selector/4 -> [CAN1_ACC_JerkUpperLimit]  "<CAN1_ACC_JerkUpperLimit>"
  [CAN1_ACC_JerkUpperLimit] -> LeftShift1/1
  LeftShift1/1 -> BitwiseAND5/1
  BitwiseAND5/1 -> [Byte_3_CAN1_ACC_JerkUpperLimit]
  bus_selector/5 -> [CAN1_ACC_RequiredAccel]  "<CAN1_ACC_RequiredAccel>"
  [CAN1_ACC_RequiredAccel] -> RightShift4/1, RightShift5/1
  RightShift4/1 -> BitwiseAND6/1
  BitwiseAND6/1 -> [Byte_1_CAN1_ACC_RequiredAccel]
  RightShift5/1 -> BitwiseAND7/1
  BitwiseAND7/1 -> [Byte_2_CAN1_ACC_RequiredAccel]
  bus_selector/6 -> [CAN1_ACC_VehHoldReq]  "<CAN1_ACC_VehHoldReq>"
  [CAN1_ACC_VehHoldReq] -> LeftShift2/1
  LeftShift2/1 -> BitwiseAND8/1
  BitwiseAND8/1 -> [Byte_0_CAN1_ACC_VehHoldReq]
  bus_selector/7 -> [CAN1_ADAS_AEBReq]  "<CAN1_ADAS_AEBReq>"
  [CAN1_ADAS_AEBReq] -> LeftShift3/1
  LeftShift3/1 -> BitwiseAND9/1
  BitwiseAND9/1 -> [Byte_1_CAN1_ADAS_AEBReq]
  bus_selector/8 -> [CAN1_ADAS_DBSReq]  "<CAN1_ADAS_DBSReq>"
  [CAN1_ADAS_DBSReq] -> LeftShift4/1
  LeftShift4/1 -> BitwiseAND10/1
  BitwiseAND10/1 -> [Byte_0_CAN1_ADAS_DBSReq]
  bus_selector/9 -> [CAN1_ADAS_FaultSta]  "<CAN1_ADAS_FaultSta>"
  [CAN1_ADAS_FaultSta] -> LeftShift5/1
  LeftShift5/1 -> BitwiseAND11/1
  BitwiseAND11/1 -> [Byte_0_CAN1_ADAS_FaultSta]
  bus_selector/10 -> [CAN1_AEB_VehHoldReq]  "<CAN1_AEB_VehHoldReq>"
  [CAN1_AEB_VehHoldReq] -> LeftShift6/1
  LeftShift6/1 -> BitwiseAND12/1
  BitwiseAND12/1 -> [Byte_0_CAN1_AEB_VehHoldReq]
  bus_selector/11 -> [CAN1_FCM2_Checksum]  "<CAN1_FCM2_Checksum>"
  [CAN1_FCM2_Checksum] -> LeftShift7/1
  LeftShift7/1 -> BitwiseAND13/1
  BitwiseAND13/1 -> [Byte_7_CAN1_FCM2_Checksum]
  bus_selector/12 -> [CAN1_FCM2_LifeCount]  "<CAN1_FCM2_LifeCount>"
  [CAN1_FCM2_LifeCount] -> LeftShift8/1
  LeftShift8/1 -> BitwiseAND14/1
  BitwiseAND14/1 -> [Byte_1_CAN1_FCM2_LifeCount]
  Data Type Conversion/1 -> BitwiseOR/1
  [Byte_0_CAN1_ACC_VehHoldReq] -> Data Type Conversion/1
  Data Type Conversion1/1 -> BitwiseOR/2
  [Byte_0_CAN1_ADAS_DBSReq] -> Data Type Conversion1/1
  Data Type Conversion2/1 -> BitwiseOR/3
  [Byte_0_CAN1_ADAS_FaultSta] -> Data Type Conversion2/1
  Data Type Conversion3/1 -> BitwiseOR/4
  [Byte_0_CAN1_AEB_VehHoldReq] -> Data Type Conversion3/1
  BitwiseOR/1 -> [Byte_0]
  Data Type Conversion4/1 -> BitwiseOR1/1
  [Byte_1_CAN1_ACC_RequiredAccel] -> Data Type Conversion4/1
  Data Type Conversion5/1 -> BitwiseOR1/2
  [Byte_1_CAN1_ADAS_AEBReq] -> Data Type Conversion5/1
  Data Type Conversion6/1 -> BitwiseOR1/3
  [Byte_1_CAN1_FCM2_LifeCount] -> Data Type Conversion6/1
  BitwiseOR1/1 -> [Byte_1]
  Data Type Conversion7/1 -> BitwiseOR2/1
  [Byte_2_CAN1_ACC_RequiredAccel] -> Data Type Conversion7/1
  BitwiseOR2/1 -> [Byte_2]
  Data Type Conversion8/1 -> BitwiseOR3/1
  [Byte_3_CAN1_ACC_ComfortBandUpper] -> Data Type Conversion8/1
  Data Type Conversion9/1 -> BitwiseOR3/2
  [Byte_3_CAN1_ACC_JerkUpperLimit] -> Data Type Conversion9/1
  BitwiseOR3/1 -> [Byte_3]
  Data Type Conversion10/1 -> BitwiseOR4/1
  [Byte_4_CAN1_ACC_ComfortBandUpper] -> Data Type Conversion10/1
  BitwiseOR4/1 -> [Byte_4]
  Data Type Conversion11/1 -> BitwiseOR5/1
  [Byte_5_CAN1_ACC_ComfortBandLower] -> Data Type Conversion11/1
  Data Type Conversion12/1 -> BitwiseOR5/2
  [Byte_5_CAN1_ACC_JerkLowerLimit] -> Data Type Conversion12/1
  BitwiseOR5/1 -> [Byte_5]
  Data Type Conversion13/1 -> BitwiseOR6/1
  [Byte_6_CAN1_ACC_ComfortBandLower] -> Data Type Conversion13/1
  BitwiseOR6/1 -> [Byte_6]
  Data Type Conversion14/1 -> BitwiseOR7/1
  [Byte_7_CAN1_FCM2_Checksum] -> Data Type Conversion14/1
  BitwiseOR7/1 -> [Byte_7]
  [Byte_0] -> Mux/1
  [Byte_1] -> Mux/2
  [Byte_2] -> Mux/3
  [Byte_3] -> Mux/4
  [Byte_4] -> Mux/5
  [Byte_5] -> Mux/6
  [Byte_6] -> Mux/7
  Mux/1 -> [VHAL_CAN1FCM2noCS_raw]
  KHAL_CAN1FCM2E2E_flg/1 -> DDM_CS&RC_Comparison/1
  0x21/1 -> DDM_CS&RC_Comparison/2
  0xb6/1 -> DDM_CS&RC_Comparison/3
  [VHAL_CAN1FCM2noCS_raw] -> DDM_CS&RC_Comparison/4
  [Byte_7] -> DDM_CS&RC_Comparison/5
  [RC_ECU] -> DDM_CS&RC_Comparison/6
  MessageRollingCounter/1 -> DDM_CS&RC_Comparison/7
  DDM_CS&RC_Comparison/1 -> VHAL_FCM2CSErr_flg/1
  DDM_CS&RC_Comparison/2 -> VHAL_FCM2RCErr_flg/1
  [DT_CAN1_SG_FCM2] -> bus_selector1/1
  bus_selector1/1 -> ACCRequiredAccel/1(ACC_RequiredAccel)  "<CAN1_ACC_RequiredAccel>"
  ACCRequiredAccel/1(VHAL_ACCRequiredAccel_mps2) -> VHAL_ACCRequiredAccel_mps2/1
  [DT_CAN1_SG_FCM2] -> bus_selector2/1
  bus_selector2/1 -> ACCVehHoldReq/1(ACC_VehHoldReq)  "<CAN1_ACC_VehHoldReq>"
  ACCVehHoldReq/1(VHAL_ACCVehHoldReq_flg) -> VHAL_ACCVehHoldReq_flg/1
  [DT_CAN1_SG_FCM2] -> bus_selector3/1
  bus_selector3/1 -> FCM2Checksum/1(FCM2_Checksum)  "<CAN1_FCM2_Checksum>"
  FCM2Checksum/1(VHAL_FCM2Checksum_enum) -> VHAL_FCM2Checksum_enum/1
  [DT_CAN1_SG_FCM2] -> bus_selector4/1
  bus_selector4/1 -> FCM2LifeCount/1(FCM2_LifeCount)  "<CAN1_FCM2_LifeCount>"
  FCM2LifeCount/1(VHAL_FCM2LifeCount_enum) -> VHAL_FCM2LifeCount_enum/1, [RC_ECU]
